simulink model "NewKitchen_demo"  (R2022b)
settings: Solver=FixedStepAuto  StartTime=0  StopTime=3*3600  FixedStep=60  RelTol=1e-3
libraries: dspswit3 x4, dspstat3 x2
settings Model: Creator=u2159176  LastModifiedBy=u2159176

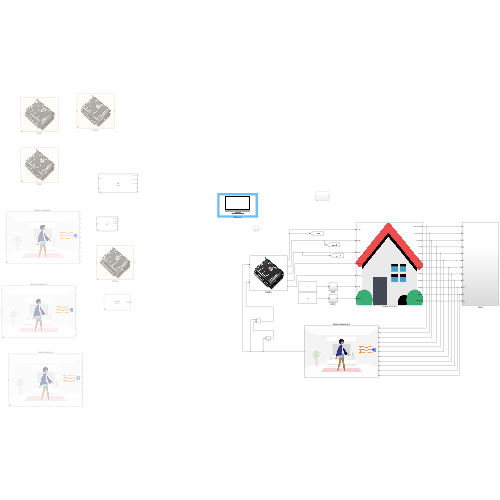
[thumbnail: Simulink's stored preview of the top-level diagram]
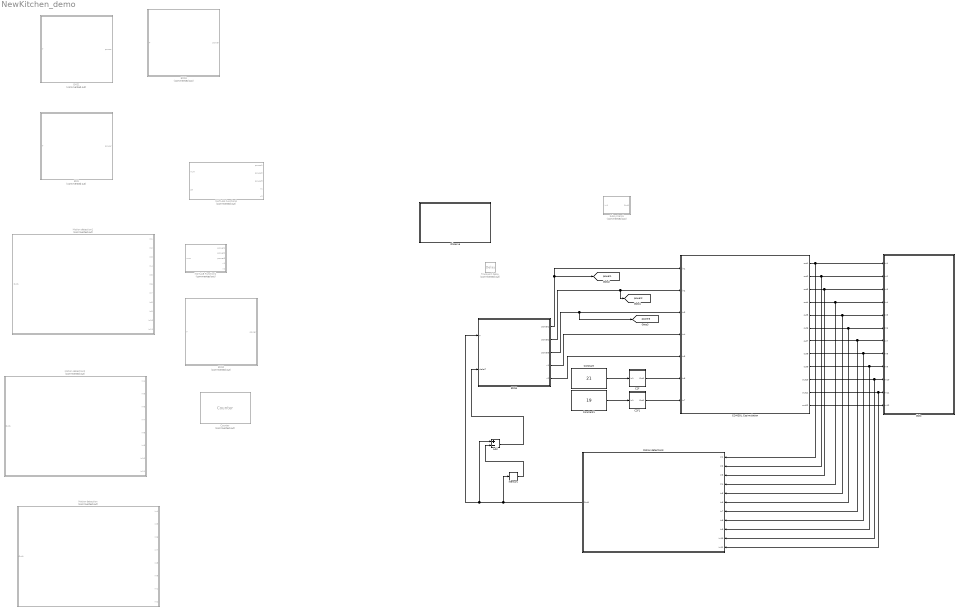
== system NewKitchen_demo ==
  Add : Sum  Inputs=+-
  C2F : Subsystem
  C2F1 : Subsystem
  COMSOL Cosimulation : Subsystem  mask(COMSOL Multiphysics Block){filename=\\brio.ads.warwick.ac.uk\User68\u\u2159176\Desktop\comsol data\ECOS2023\model1201b.fmu, dt=-1}
      mask prompts: dt "Communication step size"
      mask help: COMSOL Multiphysics Block version 6.1
      mask init:
      | if exist('cosimblockinit')==0
      |    error('Can not initialize block. Start COMSOL with Simulink and try again')
      | else
      |     cosimblockinit
      | end
      mask DialogControl bp Prompt: Block Parameters
      mask DialogControl bp Callback: setblockparameters
      mask Display:
      | if isempty(filename)
      |     root = char(java.lang.System.getProperty('cs.root'));
      |     if ~isempty(root)
      |         filename = fullfile(root, 'ext\LiveLink\Simulink\resources\llsimulink_comsol_logo_256.bmp');
      |         if exist(filename, 'file')
      |             im = imread(filename);
      |         end
      |     end
      | end
      | if exist('im', 'var')
      |     image(im)
      | else
      |     disp('COMSOL')
      | end
      | 
      | if exist('labels', 'var')
      |     if isfield(labels, 'in')
      |         for i=1:length(labels.in)
      |             port_label('input', i, labels.in{i})
      |         end
      |     end
      | 
      |     if isfield(labels, 'out')
      |         for i=1:length(labels.out)
      |             port_label('output', i, labels.out{i})
      |         end
      |     end
      | end
  Constant : Constant  Value=21
  Constant1 : Constant  Value=19
  Counter : dspswit3/Counter  Commented=on  Direction=Up  CountEvent=Free running  CounterSize=User defined  MaxCount=480  InitialCount=1  Output=Count  HitValue=1  ResetInput=off  SamplesPerFrame=1  Ts=60  CntDtype=double  HitDtype=Logical
  EMS : Stateflow chart  Commented=on  TreatAsAtomicUnit=on
  EMS1 : Stateflow chart  Commented=on  TreatAsAtomicUnit=on
  EMS2 : Stateflow chart  Commented=on  TreatAsAtomicUnit=on
  EMS3 : Stateflow chart  Commented=on  TreatAsAtomicUnit=on
  EMS4 : Stateflow chart  TreatAsAtomicUnit=on
  Goto : Subsystem
  MATLAB Function1 : MATLAB Function  Commented=on  TreatAsAtomicUnit=on
  MATLAB Function3 : MATLAB Function  Commented=on  TreatAsAtomicUnit=on
  Memory : Memory
  Motion detection : Subsystem  Commented=on
      mask Display: image('\\brio.ads.warwick.ac.uk\User68\u\u2159176\Desktop\comsol data\ECOS2023\tanshen\microwave-sensor.jpg'); % Use "Edit Image" on toolstrip to change.
  Motion detection1 : Subsystem  Commented=on
      mask Display: image('\\brio.ads.warwick.ac.uk\User68\u\u2159176\Desktop\comsol data\ECOS2023\tanshen\microwave-sensor.jpg'); % Use "Edit Image" on toolstrip to change.
  Motion detection2 : Subsystem  Commented=on
      mask Display: image('\\brio.ads.warwick.ac.uk\User68\u\u2159176\Desktop\comsol data\ECOS2023\tanshen\microwave-sensor.jpg'); % Use "Edit Image" on toolstrip to change.
  Motion detection3 : Subsystem
      mask Display: image('\\brio.ads.warwick.ac.uk\User68\u\u2159176\Desktop\comsol data\ECOS2023\tanshen\microwave-sensor.jpg'); % Use "Edit Image" on toolstrip to change.
  Observe : Subsystem
      mask Display: image('\\brio.ads.warwick.ac.uk\User68\u\u2159176\Desktop\comsol data\ECOS2023\tanshen\lcd_display.png'); % Use "Edit Image" on toolstrip to change.
  Subsystem5 : Subsystem  Commented=on
  Transport Delay : TransportDelay  Commented=on
  tag scope: power1=global, power2=global, power3=global
  wires:
  Constant/1 -> C2F/1(In1)
  Constant1/1 -> C2F1/1(In1)
  COMSOL Cosimulation/1(out1) -> Motion detection3/1(In1), Goto/1(In1)
  COMSOL Cosimulation/2(out2) -> Motion detection3/2(In2), Goto/2(In2)
  COMSOL Cosimulation/3(out3) -> Motion detection3/3(In3), Goto/3(In3)
  COMSOL Cosimulation/4(out4) -> Motion detection3/4(In4), Goto/4(In4)
  COMSOL Cosimulation/5(out5) -> Motion detection3/5(In5), Goto/5(In5)
  COMSOL Cosimulation/6(out6) -> Motion detection3/6(In6), Goto/6(In6)
  COMSOL Cosimulation/7(out7) -> Motion detection3/7(In7), Goto/7(In7)
  COMSOL Cosimulation/8(out8) -> Motion detection3/8(In8), Goto/8(In8)
  COMSOL Cosimulation/9(out9) -> Motion detection3/9(In9), Goto/9(In9)
  COMSOL Cosimulation/10(out10) -> Motion detection3/10(In10), Goto/10(In10)
  COMSOL Cosimulation/11(out11) -> Motion detection3/11(In11), Goto/11(In11)
  COMSOL Cosimulation/12(out12) -> Goto/12(In12)
  C2F/1(Out1) -> COMSOL Cosimulation/6(in6)
  C2F1/1(Out1) -> COMSOL Cosimulation/7(in7)
  Motion detection3/1(Out1) -> Add/1, EMS4/1(T), Memory/1
  Memory/1 -> Add/2
  Add/1 -> EMS4/2(deltaT)
  EMS4/1(power1) -> COMSOL Cosimulation/1(in1), [power1]
  EMS4/2(power2) -> [power2], COMSOL Cosimulation/2(in2)
  EMS4/3(power3) -> [power3], COMSOL Cosimulation/3(in3)
  EMS4/4(v1) -> COMSOL Cosimulation/4(in4)
  EMS4/5(v2) -> COMSOL Cosimulation/5(in5)

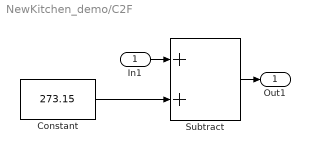
== system NewKitchen_demo/C2F ==
  In1 : Inport
  Constant : Constant  Value=273.15
  Subtract : Sum
  Out1 : Outport
  wires:
  In1/1 -> Subtract/1
  Constant/1 -> Subtract/2
  Subtract/1 -> Out1/1

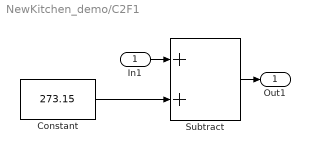
== system NewKitchen_demo/C2F1 ==
  In1 : Inport
  Constant : Constant  Value=273.15
  Subtract : Sum
  Out1 : Outport
  wires:
  Subtract/1 -> Out1/1
  Constant/1 -> Subtract/2
  In1/1 -> Subtract/1

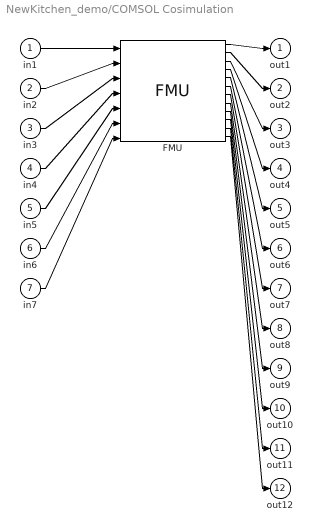
== system NewKitchen_demo/COMSOL Cosimulation ==
  in1 : Inport
  in2 : Inport  Port=2
  in3 : Inport  Port=3
  in4 : Inport  Port=4
  in5 : Inport  Port=5
  in6 : Inport  Port=6
  in7 : Inport  Port=7
  FMU : FMU  FMUName=model1201b.fmu  FMUDebugLogging=on  FMUMode=CoSimulation
      mask Type: demo1122bfor61.mph [Co-Simulation, v2.0]
      mask Display:
      | if (exist([Simulink.fileGenControl('get','CacheFolder') '\slprj\_fmu\ac9248b5f738903d145a6e09f814e397\model1201b\model.png'],'file'))
      |     image([Simulink.fileGenControl('get','CacheFolder') '\slprj\_fmu\ac9248b5f738903d145a6e09f814e397\model1201b\model.png']);
      | else
      |     disp('demo1122bfor61.mph');
      | end
      | port_label('output',1,'comp1.point1');
      | port_label('output',2,'comp1.point2');
      | port_label('output',3,'comp1.point3');
      | port_label('output',4,'comp1.edge1');
      | port_label('output',5,'comp1.edge2');
      | port_label('output',6,'comp1.edge3');
      | port_label('output',7,'comp1.edge4');
      | port_label('output',8,'comp1.edge5');
      | port_label('output',9,'comp1.edge6');
      | port_label('output',10,'comp1.edge7');
      | port_label('output',11,'comp1.edge8');
      | port_label('output',12,'comp1.dom1');
      | port_label('input',1,'P1');
      | port_label('input',2,'P2');
      | port_label('input',3,'P3');
      | port_label('input',4,'V1');
      | port_label('input',5,'V2');
      | port_label('input',6,'Tin');
      | port_label('input',7,'Tout');
  out1 : Outport
  out2 : Outport  Port=2
  out3 : Outport  Port=3
  out4 : Outport  Port=4
  out5 : Outport  Port=5
  out6 : Outport  Port=6
  out7 : Outport  Port=7
  out8 : Outport  Port=8
  out9 : Outport  Port=9
  out10 : Outport  Port=10
  out11 : Outport  Port=11
  out12 : Outport  Port=12
  wires:
  FMU/1 -> out1/1
  FMU/2 -> out2/1
  FMU/3 -> out3/1
  FMU/4 -> out4/1
  FMU/5 -> out5/1
  FMU/6 -> out6/1
  FMU/7 -> out7/1
  FMU/8 -> out8/1
  FMU/9 -> out9/1
  FMU/10 -> out10/1
  FMU/11 -> out11/1
  FMU/12 -> out12/1
  in1/1 -> FMU/1
  in2/1 -> FMU/2
  in3/1 -> FMU/3
  in4/1 -> FMU/4
  in5/1 -> FMU/5
  in6/1 -> FMU/6
  in7/1 -> FMU/7

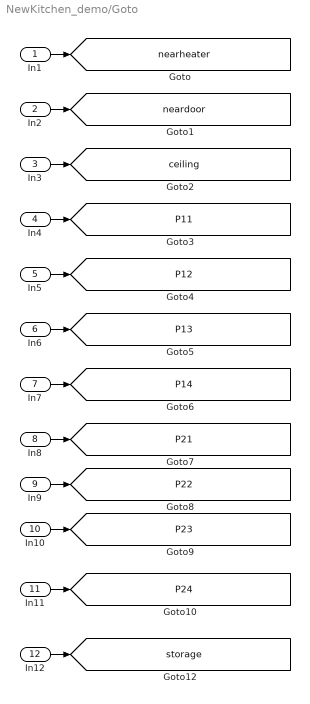
== system NewKitchen_demo/Goto ==
  In1 : Inport
  In2 : Inport  Port=2
  In3 : Inport  Port=3
  In4 : Inport  Port=4
  In5 : Inport  Port=5
  In6 : Inport  Port=6
  In7 : Inport  Port=7
  In8 : Inport  Port=8
  In9 : Inport  Port=9
  In10 : Inport  Port=10
  In11 : Inport  Port=11
  In12 : Inport  Port=12
  tag scope: P11=global, P12=global, P13=global, P14=global, P21=global, P22=global, P23=global, P24=global, ceiling=global, neardoor=global, nearheater=global, storage=global
  wires:
  In2/1 -> [neardoor]
  In10/1 -> [P23]
  In4/1 -> [P11]
  In3/1 -> [ceiling]
  In11/1 -> [P24]
  In8/1 -> [P21]
  In7/1 -> [P14]
  In5/1 -> [P12]
  In6/1 -> [P13]
  In1/1 -> [nearheater]
  In9/1 -> [P22]
  In12/1 -> [storage]

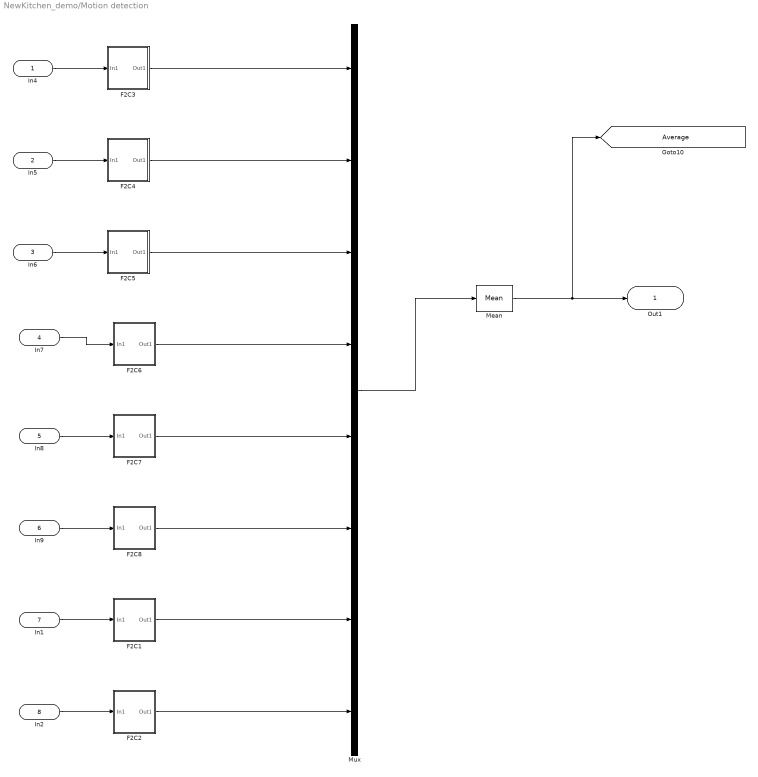
== system NewKitchen_demo/Motion detection ==
  In4 : Inport
  In5 : Inport  Port=2
  In6 : Inport  Port=3
  In7 : Inport  Port=4
  In8 : Inport  Port=5
  In9 : Inport  Port=6
  In1 : Inport  Port=7
  In2 : Inport  Port=8
  F2C1 : Subsystem
  F2C2 : Subsystem
  F2C3 : Subsystem
  F2C4 : Subsystem
  F2C5 : Subsystem
  F2C6 : Subsystem
  F2C7 : Subsystem
  F2C8 : Subsystem
  Mean : dspstat3/Mean  run=off  InputProcessing=Columns as channels (frame based)  reset_popup=None  directionMode=Each column  dimension=1  roiEnable=off  roiType=Rectangles  roiPortion=Entire ROI  roiOutput=Individual statistics for each ROI  roiFlag=off  roundingMode=Floor  overflowMode=off  outputDataTypeStr=Inherit: Same as accumulator  outputMin=[]  outputMax=[]  outputLastDataTypeStr=Inherit: Same as accumulator
  Mux : Mux  Inputs=8
  Out1 : Outport
  tag scope: Average=global
  wires:
  In4/1 -> F2C3/1(In1)
  In5/1 -> F2C4/1(In1)
  In6/1 -> F2C5/1(In1)
  In7/1 -> F2C6/1(In1)
  In8/1 -> F2C7/1(In1)
  In9/1 -> F2C8/1(In1)
  Mean/1 -> [Average], Out1/1
  Mux/1 -> Mean/1
  F2C3/1(Out1) -> Mux/1
  F2C4/1(Out1) -> Mux/2
  F2C5/1(Out1) -> Mux/3
  F2C6/1(Out1) -> Mux/4
  F2C7/1(Out1) -> Mux/5
  F2C8/1(Out1) -> Mux/6
  F2C1/1(Out1) -> Mux/7
  In1/1 -> F2C1/1(In1)
  In2/1 -> F2C2/1(In1)
  F2C2/1(Out1) -> Mux/8

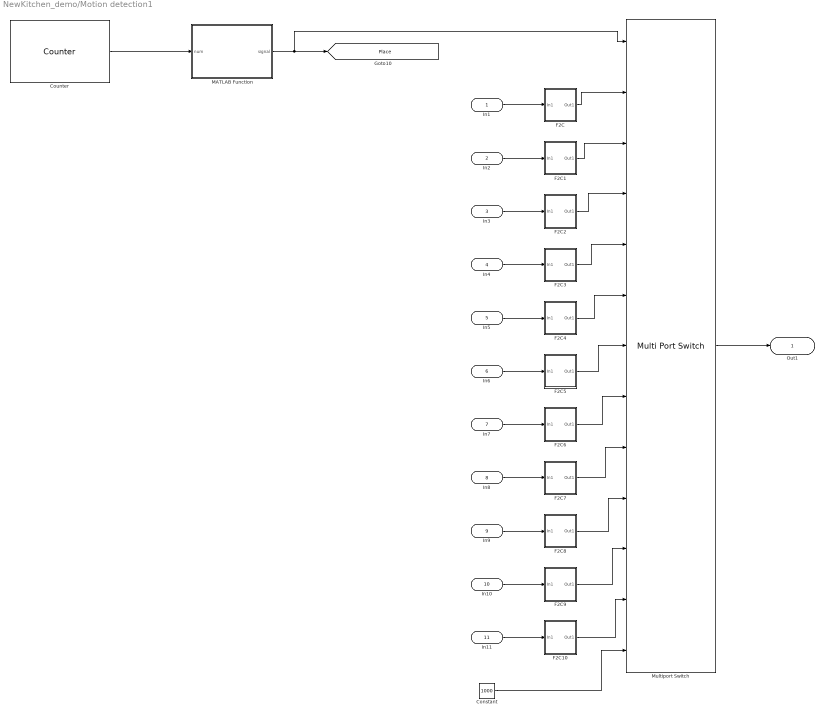
== system NewKitchen_demo/Motion detection1 ==
  In1 : Inport
  In2 : Inport  Port=2
  In3 : Inport  Port=3
  In4 : Inport  Port=4
  In5 : Inport  Port=5
  In6 : Inport  Port=6
  In7 : Inport  Port=7
  In8 : Inport  Port=8
  In9 : Inport  Port=9
  In10 : Inport  Port=10
  In11 : Inport  Port=11
  Constant : Constant  Value=1000
  Counter : dspswit3/Counter  Direction=Up  CountEvent=Free running  CounterSize=User defined  MaxCount=480  InitialCount=1  Output=Count  HitValue=1  ResetInput=off  SamplesPerFrame=1  Ts=60  CntDtype=double  HitDtype=Logical
  F2C : Subsystem
  F2C1 : Subsystem
  F2C10 : Subsystem
  F2C2 : Subsystem
  F2C3 : Subsystem
  F2C4 : Subsystem
  F2C5 : Subsystem
  F2C6 : Subsystem
  F2C7 : Subsystem
  F2C8 : Subsystem
  F2C9 : Subsystem
  MATLAB Function : MATLAB Function  TreatAsAtomicUnit=on
  Multiport Switch : MultiPortSwitch  Inputs=12  SaturateOnIntegerOverflow=off  InputSameDT=off
  Out1 : Outport
  tag scope: Place=global
  wires:
  Constant/1 -> Multiport Switch/13
  MATLAB Function/1(signal) -> [Place], Multiport Switch/1
  Counter/1 -> MATLAB Function/1(num)
  Multiport Switch/1 -> Out1/1
  In11/1 -> F2C10/1(In1)
  In10/1 -> F2C9/1(In1)
  In9/1 -> F2C8/1(In1)
  In8/1 -> F2C7/1(In1)
  In7/1 -> F2C6/1(In1)
  In6/1 -> F2C5/1(In1)
  In5/1 -> F2C4/1(In1)
  In4/1 -> F2C3/1(In1)
  In3/1 -> F2C2/1(In1)
  In2/1 -> F2C1/1(In1)
  In1/1 -> F2C/1(In1)
  F2C10/1(Out1) -> Multiport Switch/12
  F2C9/1(Out1) -> Multiport Switch/11
  F2C8/1(Out1) -> Multiport Switch/10
  F2C7/1(Out1) -> Multiport Switch/9
  F2C6/1(Out1) -> Multiport Switch/8
  F2C5/1(Out1) -> Multiport Switch/7
  F2C4/1(Out1) -> Multiport Switch/6
  F2C3/1(Out1) -> Multiport Switch/5
  F2C2/1(Out1) -> Multiport Switch/4
  F2C1/1(Out1) -> Multiport Switch/3
  F2C/1(Out1) -> Multiport Switch/2

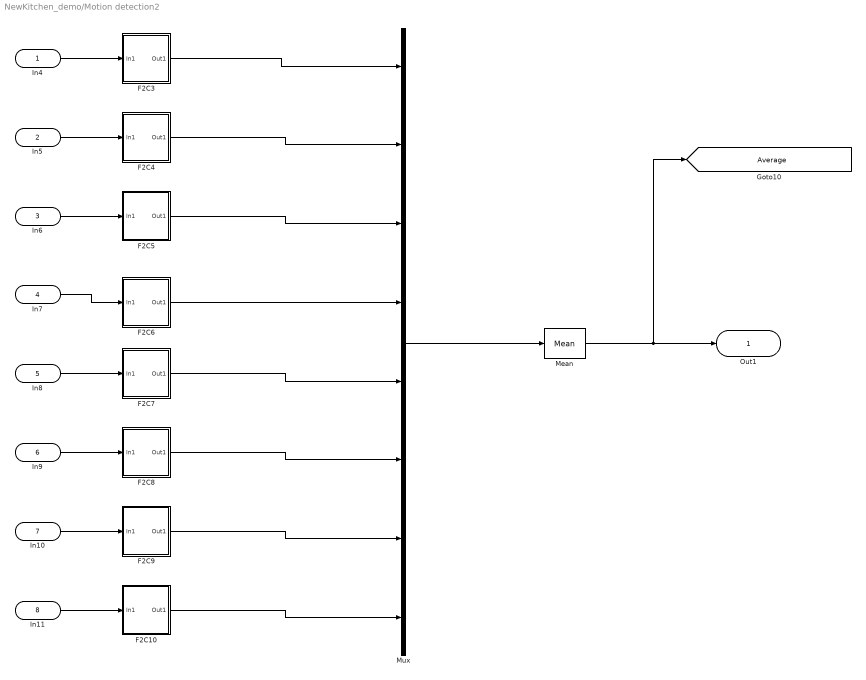
== system NewKitchen_demo/Motion detection2 ==
  In4 : Inport
  In5 : Inport  Port=2
  In6 : Inport  Port=3
  In7 : Inport  Port=4
  In8 : Inport  Port=5
  In9 : Inport  Port=6
  In10 : Inport  Port=7
  In11 : Inport  Port=8
  F2C10 : Subsystem
  F2C3 : Subsystem
  F2C4 : Subsystem
  F2C5 : Subsystem
  F2C6 : Subsystem
  F2C7 : Subsystem
  F2C8 : Subsystem
  F2C9 : Subsystem
  Mean : dspstat3/Mean  run=off  InputProcessing=Columns as channels (frame based)  reset_popup=None  directionMode=Each column  dimension=1  roiEnable=off  roiType=Rectangles  roiPortion=Entire ROI  roiOutput=Individual statistics for each ROI  roiFlag=off  roundingMode=Floor  overflowMode=off  outputDataTypeStr=Inherit: Same as accumulator  outputMin=[]  outputMax=[]  outputLastDataTypeStr=Inherit: Same as accumulator
  Mux : Mux  Inputs=8
  Out1 : Outport
  tag scope: Average=global
  wires:
  F2C10/1(Out1) -> Mux/8
  F2C9/1(Out1) -> Mux/7
  F2C8/1(Out1) -> Mux/6
  F2C7/1(Out1) -> Mux/5
  F2C6/1(Out1) -> Mux/4
  F2C5/1(Out1) -> Mux/3
  F2C4/1(Out1) -> Mux/2
  F2C3/1(Out1) -> Mux/1
  Mux/1 -> Mean/1
  Mean/1 -> Out1/1, [Average]
  In11/1 -> F2C10/1(In1)
  In10/1 -> F2C9/1(In1)
  In9/1 -> F2C8/1(In1)
  In8/1 -> F2C7/1(In1)
  In7/1 -> F2C6/1(In1)
  In6/1 -> F2C5/1(In1)
  In5/1 -> F2C4/1(In1)
  In4/1 -> F2C3/1(In1)

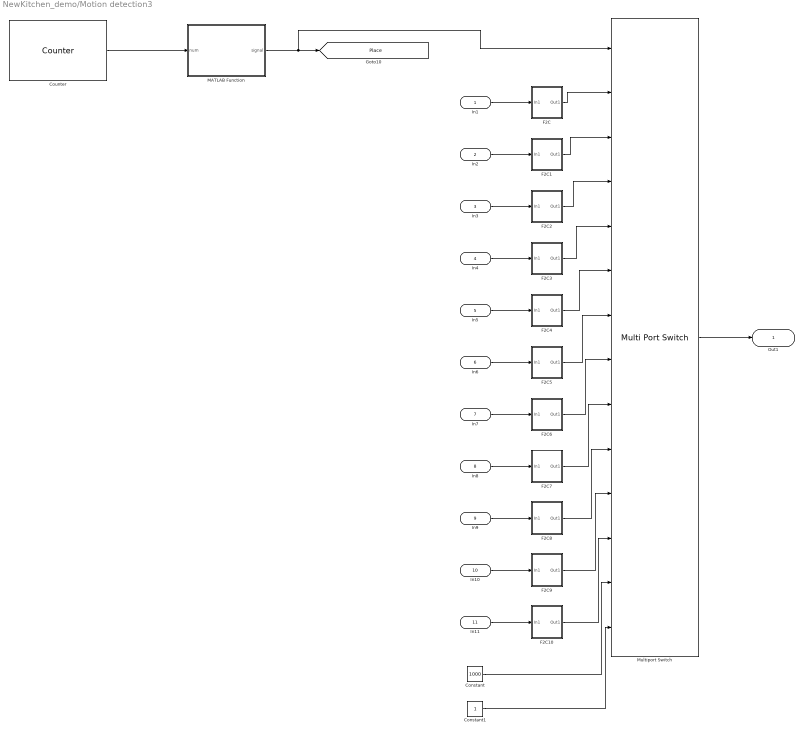
== system NewKitchen_demo/Motion detection3 ==
  In1 : Inport
  In2 : Inport  Port=2
  In3 : Inport  Port=3
  In4 : Inport  Port=4
  In5 : Inport  Port=5
  In6 : Inport  Port=6
  In7 : Inport  Port=7
  In8 : Inport  Port=8
  In9 : Inport  Port=9
  In10 : Inport  Port=10
  In11 : Inport  Port=11
  Constant : Constant  Value=1000
  Constant1 : Constant
  Counter : dspswit3/Counter  Direction=Up  CountEvent=Free running  CounterSize=User defined  MaxCount=480  InitialCount=1  Output=Count  HitValue=1  ResetInput=off  SamplesPerFrame=1  Ts=60  CntDtype=double  HitDtype=Logical
  F2C : Subsystem
  F2C1 : Subsystem
  F2C10 : Subsystem
  F2C2 : Subsystem
  F2C3 : Subsystem
  F2C4 : Subsystem
  F2C5 : Subsystem
  F2C6 : Subsystem
  F2C7 : Subsystem
  F2C8 : Subsystem
  F2C9 : Subsystem
  MATLAB Function : MATLAB Function  TreatAsAtomicUnit=on
  Multiport Switch : MultiPortSwitch  Inputs=13  SaturateOnIntegerOverflow=off  InputSameDT=off
  Out1 : Outport
  tag scope: Place=global
  wires:
  F2C/1(Out1) -> Multiport Switch/2
  F2C1/1(Out1) -> Multiport Switch/3
  F2C2/1(Out1) -> Multiport Switch/4
  F2C3/1(Out1) -> Multiport Switch/5
  F2C4/1(Out1) -> Multiport Switch/6
  F2C5/1(Out1) -> Multiport Switch/7
  F2C6/1(Out1) -> Multiport Switch/8
  F2C7/1(Out1) -> Multiport Switch/9
  F2C8/1(Out1) -> Multiport Switch/10
  F2C9/1(Out1) -> Multiport Switch/11
  F2C10/1(Out1) -> Multiport Switch/12
  In1/1 -> F2C/1(In1)
  In2/1 -> F2C1/1(In1)
  In3/1 -> F2C2/1(In1)
  In4/1 -> F2C3/1(In1)
  In5/1 -> F2C4/1(In1)
  In6/1 -> F2C5/1(In1)
  In7/1 -> F2C6/1(In1)
  In8/1 -> F2C7/1(In1)
  In9/1 -> F2C8/1(In1)
  In10/1 -> F2C9/1(In1)
  In11/1 -> F2C10/1(In1)
  Multiport Switch/1 -> Out1/1
  Counter/1 -> MATLAB Function/1(num)
  MATLAB Function/1(signal) -> Multiport Switch/1, [Place]
  Constant/1 -> Multiport Switch/13
  Constant1/1 -> Multiport Switch/14

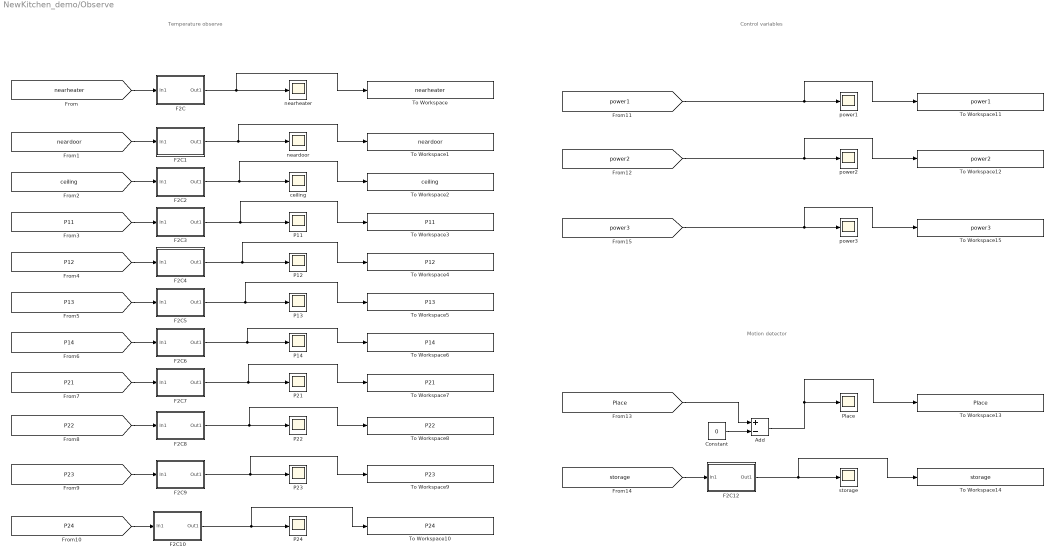
== system NewKitchen_demo/Observe ==
  note: Temperature observe
  note: Control variables
  note: Motion detector
  Add : Sum  Inputs=+-
  Constant : Constant  Value=0
  F2C : Subsystem
  F2C1 : Subsystem
  F2C10 : Subsystem
  F2C12 : Subsystem
  F2C2 : Subsystem
  F2C3 : Subsystem
  F2C4 : Subsystem
  F2C5 : Subsystem
  F2C6 : Subsystem
  F2C7 : Subsystem
  F2C8 : Subsystem
  F2C9 : Subsystem
  P{11..14,21..24} (8 alike) : Scope
  Place : Scope
  To Workspace : ToWorkspace  VariableName=nearheater  SampleTime=-1
  To Workspace1 : ToWorkspace  VariableName=neardoor  SampleTime=-1
  To Workspace10 : ToWorkspace  VariableName=P24  SampleTime=-1
  To Workspace11 : ToWorkspace  VariableName=power1  SampleTime=-1
  To Workspace12 : ToWorkspace  VariableName=power2  SampleTime=-1
  To Workspace13 : ToWorkspace  VariableName=Place  SampleTime=-1
  To Workspace14 : ToWorkspace  VariableName=storage  SampleTime=-1
  To Workspace15 : ToWorkspace  VariableName=power3  SampleTime=-1
  To Workspace2 : ToWorkspace  VariableName=ceiling  SampleTime=-1
  To Workspace3 : ToWorkspace  VariableName=P11  SampleTime=-1
  To Workspace4 : ToWorkspace  VariableName=P12  SampleTime=-1
  To Workspace5 : ToWorkspace  VariableName=P13  SampleTime=-1
  To Workspace6 : ToWorkspace  VariableName=P14  SampleTime=-1
  To Workspace7 : ToWorkspace  VariableName=P21  SampleTime=-1
  To Workspace8 : ToWorkspace  VariableName=P22  SampleTime=-1
  To Workspace9 : ToWorkspace  VariableName=P23  SampleTime=-1
  ceiling : Scope
  neardoor : Scope
  nearheater : Scope
  power1 : Scope
  power2 : Scope
  power3 : Scope
  storage : Scope
  wires:
  [nearheater] -> F2C/1(In1)
  F2C/1(Out1) -> To Workspace/1, nearheater/1
  [neardoor] -> F2C1/1(In1)
  F2C1/1(Out1) -> To Workspace1/1, neardoor/1
  [ceiling] -> F2C2/1(In1)
  F2C2/1(Out1) -> To Workspace2/1, ceiling/1
  [P11] -> F2C3/1(In1)
  F2C3/1(Out1) -> To Workspace3/1, P11/1
  [P12] -> F2C4/1(In1)
  F2C4/1(Out1) -> To Workspace4/1, P12/1
  [P13] -> F2C5/1(In1)
  F2C5/1(Out1) -> To Workspace5/1, P13/1
  [P14] -> F2C6/1(In1)
  F2C6/1(Out1) -> To Workspace6/1, P14/1
  [P21] -> F2C7/1(In1)
  F2C7/1(Out1) -> To Workspace7/1, P21/1
  [P22] -> F2C8/1(In1)
  F2C8/1(Out1) -> To Workspace8/1, P22/1
  [P23] -> F2C9/1(In1)
  F2C9/1(Out1) -> To Workspace9/1, P23/1
  [P24] -> F2C10/1(In1)
  [power1] -> To Workspace11/1, power1/1
  F2C10/1(Out1) -> To Workspace10/1, P24/1
  F2C12/1(Out1) -> storage/1, To Workspace14/1
  [storage] -> F2C12/1(In1)
  [power2] -> power2/1, To Workspace12/1
  [power3] -> To Workspace15/1, power3/1
  Constant/1 -> Add/2
  [Place] -> Add/1
  Add/1 -> To Workspace13/1, Place/1

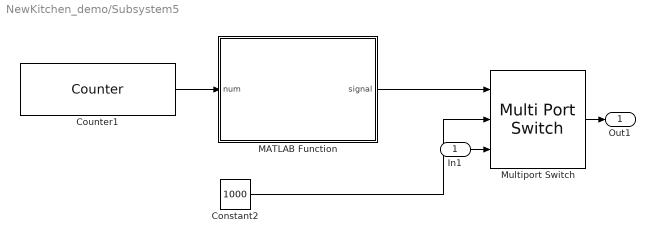
== system NewKitchen_demo/Subsystem5 ==
  In1 : Inport
  Constant2 : Constant  Value=1000
  Counter1 : dspswit3/Counter  Direction=Up  CountEvent=Free running  CounterSize=User defined  MaxCount=480  InitialCount=1  Output=Count  HitValue=1  ResetInput=off  SamplesPerFrame=1  Ts=60  CntDtype=double  HitDtype=Logical
  MATLAB Function : MATLAB Function  TreatAsAtomicUnit=on
  Multiport Switch : MultiPortSwitch  Inputs=2  SaturateOnIntegerOverflow=off  InputSameDT=off
  Out1 : Outport
  wires:
  Multiport Switch/1 -> Out1/1
  Constant2/1 -> Multiport Switch/2
  MATLAB Function/1(signal) -> Multiport Switch/1
  In1/1 -> Multiport Switch/3
  Counter1/1 -> MATLAB Function/1(num)

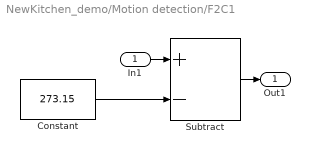
== system NewKitchen_demo/Motion detection/F2C1 ==
  In1 : Inport
  Constant : Constant  Value=273.15
  Subtract : Sum  Inputs=+-
  Out1 : Outport
  wires:
  Subtract/1 -> Out1/1
  Constant/1 -> Subtract/2
  In1/1 -> Subtract/1

== system NewKitchen_demo/Motion detection/F2C2 ==
  In1 : Inport
  Constant : Constant  Value=273.15
  Subtract : Sum  Inputs=+-
  Out1 : Outport
  wires:
  In1/1 -> Subtract/1
  Constant/1 -> Subtract/2
  Subtract/1 -> Out1/1

== system NewKitchen_demo/Motion detection/F2C3 ==
  In1 : Inport
  Constant : Constant  Value=273.15
  Subtract : Sum  Inputs=+-
  Out1 : Outport
  wires:
  Subtract/1 -> Out1/1
  Constant/1 -> Subtract/2
  In1/1 -> Subtract/1

== system NewKitchen_demo/Motion detection/F2C4 ==
  In1 : Inport
  Constant : Constant  Value=273.15
  Subtract : Sum  Inputs=+-
  Out1 : Outport
  wires:
  In1/1 -> Subtract/1
  Constant/1 -> Subtract/2
  Subtract/1 -> Out1/1

== system NewKitchen_demo/Motion detection/F2C5 ==
  In1 : Inport
  Constant : Constant  Value=273.15
  Subtract : Sum  Inputs=+-
  Out1 : Outport
  wires:
  Subtract/1 -> Out1/1
  Constant/1 -> Subtract/2
  In1/1 -> Subtract/1

== system NewKitchen_demo/Motion detection/F2C6 ==
  In1 : Inport
  Constant : Constant  Value=273.15
  Subtract : Sum  Inputs=+-
  Out1 : Outport
  wires:
  In1/1 -> Subtract/1
  Constant/1 -> Subtract/2
  Subtract/1 -> Out1/1

== system NewKitchen_demo/Motion detection/F2C7 ==
  In1 : Inport
  Constant : Constant  Value=273.15
  Subtract : Sum  Inputs=+-
  Out1 : Outport
  wires:
  Subtract/1 -> Out1/1
  Constant/1 -> Subtract/2
  In1/1 -> Subtract/1

== system NewKitchen_demo/Motion detection/F2C8 ==
  In1 : Inport
  Constant : Constant  Value=273.15
  Subtract : Sum  Inputs=+-
  Out1 : Outport
  wires:
  In1/1 -> Subtract/1
  Constant/1 -> Subtract/2
  Subtract/1 -> Out1/1

== system NewKitchen_demo/Motion detection1/F2C ==
  In1 : Inport
  Constant : Constant  Value=273.15
  Subtract : Sum  Inputs=+-
  Out1 : Outport
  wires:
  Subtract/1 -> Out1/1
  Constant/1 -> Subtract/2
  In1/1 -> Subtract/1

== system NewKitchen_demo/Motion detection1/F2C1 ==
  In1 : Inport
  Constant : Constant  Value=273.15
  Subtract : Sum  Inputs=+-
  Out1 : Outport
  wires:
  In1/1 -> Subtract/1
  Constant/1 -> Subtract/2
  Subtract/1 -> Out1/1

== system NewKitchen_demo/Motion detection1/F2C10 ==
  In1 : Inport
  Constant : Constant  Value=273.15
  Subtract : Sum  Inputs=+-
  Out1 : Outport
  wires:
  Subtract/1 -> Out1/1
  Constant/1 -> Subtract/2
  In1/1 -> Subtract/1

== system NewKitchen_demo/Motion detection1/F2C2 ==
  In1 : Inport
  Constant : Constant  Value=273.15
  Subtract : Sum  Inputs=+-
  Out1 : Outport
  wires:
  Subtract/1 -> Out1/1
  Constant/1 -> Subtract/2
  In1/1 -> Subtract/1

== system NewKitchen_demo/Motion detection1/F2C3 ==
  In1 : Inport
  Constant : Constant  Value=273.15
  Subtract : Sum  Inputs=+-
  Out1 : Outport
  wires:
  In1/1 -> Subtract/1
  Constant/1 -> Subtract/2
  Subtract/1 -> Out1/1

== system NewKitchen_demo/Motion detection1/F2C4 ==
  In1 : Inport
  Constant : Constant  Value=273.15
  Subtract : Sum  Inputs=+-
  Out1 : Outport
  wires:
  Subtract/1 -> Out1/1
  Constant/1 -> Subtract/2
  In1/1 -> Subtract/1

== system NewKitchen_demo/Motion detection1/F2C5 ==
  In1 : Inport
  Constant : Constant  Value=273.15
  Subtract : Sum  Inputs=+-
  Out1 : Outport
  wires:
  In1/1 -> Subtract/1
  Constant/1 -> Subtract/2
  Subtract/1 -> Out1/1

== system NewKitchen_demo/Motion detection1/F2C6 ==
  In1 : Inport
  Constant : Constant  Value=273.15
  Subtract : Sum  Inputs=+-
  Out1 : Outport
  wires:
  Subtract/1 -> Out1/1
  Constant/1 -> Subtract/2
  In1/1 -> Subtract/1

== system NewKitchen_demo/Motion detection1/F2C7 ==
  In1 : Inport
  Constant : Constant  Value=273.15
  Subtract : Sum  Inputs=+-
  Out1 : Outport
  wires:
  In1/1 -> Subtract/1
  Constant/1 -> Subtract/2
  Subtract/1 -> Out1/1

== system NewKitchen_demo/Motion detection1/F2C8 ==
  In1 : Inport
  Constant : Constant  Value=273.15
  Subtract : Sum  Inputs=+-
  Out1 : Outport
  wires:
  Subtract/1 -> Out1/1
  Constant/1 -> Subtract/2
  In1/1 -> Subtract/1

== system NewKitchen_demo/Motion detection1/F2C9 ==
  In1 : Inport
  Constant : Constant  Value=273.15
  Subtract : Sum  Inputs=+-
  Out1 : Outport
  wires:
  In1/1 -> Subtract/1
  Constant/1 -> Subtract/2
  Subtract/1 -> Out1/1

== system NewKitchen_demo/Motion detection2/F2C10 ==
  In1 : Inport
  Constant : Constant  Value=273.15
  Subtract : Sum  Inputs=+-
  Out1 : Outport
  wires:
  Subtract/1 -> Out1/1
  Constant/1 -> Subtract/2
  In1/1 -> Subtract/1

== system NewKitchen_demo/Motion detection2/F2C3 ==
  In1 : Inport
  Constant : Constant  Value=273.15
  Subtract : Sum  Inputs=+-
  Out1 : Outport
  wires:
  In1/1 -> Subtract/1
  Constant/1 -> Subtract/2
  Subtract/1 -> Out1/1

== system NewKitchen_demo/Motion detection2/F2C4 ==
  In1 : Inport
  Constant : Constant  Value=273.15
  Subtract : Sum  Inputs=+-
  Out1 : Outport
  wires:
  Subtract/1 -> Out1/1
  Constant/1 -> Subtract/2
  In1/1 -> Subtract/1

== system NewKitchen_demo/Motion detection2/F2C5 ==
  In1 : Inport
  Constant : Constant  Value=273.15
  Subtract : Sum  Inputs=+-
  Out1 : Outport
  wires:
  In1/1 -> Subtract/1
  Constant/1 -> Subtract/2
  Subtract/1 -> Out1/1

== system NewKitchen_demo/Motion detection2/F2C6 ==
  In1 : Inport
  Constant : Constant  Value=273.15
  Subtract : Sum  Inputs=+-
  Out1 : Outport
  wires:
  Subtract/1 -> Out1/1
  Constant/1 -> Subtract/2
  In1/1 -> Subtract/1

== system NewKitchen_demo/Motion detection2/F2C7 ==
  In1 : Inport
  Constant : Constant  Value=273.15
  Subtract : Sum  Inputs=+-
  Out1 : Outport
  wires:
  In1/1 -> Subtract/1
  Constant/1 -> Subtract/2
  Subtract/1 -> Out1/1

== system NewKitchen_demo/Motion detection2/F2C8 ==
  In1 : Inport
  Constant : Constant  Value=273.15
  Subtract : Sum  Inputs=+-
  Out1 : Outport
  wires:
  Subtract/1 -> Out1/1
  Constant/1 -> Subtract/2
  In1/1 -> Subtract/1

== system NewKitchen_demo/Motion detection2/F2C9 ==
  In1 : Inport
  Constant : Constant  Value=273.15
  Subtract : Sum  Inputs=+-
  Out1 : Outport
  wires:
  In1/1 -> Subtract/1
  Constant/1 -> Subtract/2
  Subtract/1 -> Out1/1

== system NewKitchen_demo/Motion detection3/F2C ==
  In1 : Inport
  Constant : Constant  Value=273.15
  Subtract : Sum  Inputs=+-
  Out1 : Outport
  wires:
  In1/1 -> Subtract/1
  Constant/1 -> Subtract/2
  Subtract/1 -> Out1/1

== system NewKitchen_demo/Motion detection3/F2C1 ==
  In1 : Inport
  Constant : Constant  Value=273.15
  Subtract : Sum  Inputs=+-
  Out1 : Outport
  wires:
  Subtract/1 -> Out1/1
  Constant/1 -> Subtract/2
  In1/1 -> Subtract/1

== system NewKitchen_demo/Motion detection3/F2C10 ==
  In1 : Inport
  Constant : Constant  Value=273.15
  Subtract : Sum  Inputs=+-
  Out1 : Outport
  wires:
  In1/1 -> Subtract/1
  Constant/1 -> Subtract/2
  Subtract/1 -> Out1/1

== system NewKitchen_demo/Motion detection3/F2C2 ==
  In1 : Inport
  Constant : Constant  Value=273.15
  Subtract : Sum  Inputs=+-
  Out1 : Outport
  wires:
  In1/1 -> Subtract/1
  Constant/1 -> Subtract/2
  Subtract/1 -> Out1/1

== system NewKitchen_demo/Motion detection3/F2C3 ==
  In1 : Inport
  Constant : Constant  Value=273.15
  Subtract : Sum  Inputs=+-
  Out1 : Outport
  wires:
  Subtract/1 -> Out1/1
  Constant/1 -> Subtract/2
  In1/1 -> Subtract/1

== system NewKitchen_demo/Motion detection3/F2C4 ==
  In1 : Inport
  Constant : Constant  Value=273.15
  Subtract : Sum  Inputs=+-
  Out1 : Outport
  wires:
  In1/1 -> Subtract/1
  Constant/1 -> Subtract/2
  Subtract/1 -> Out1/1

== system NewKitchen_demo/Motion detection3/F2C5 ==
  In1 : Inport
  Constant : Constant  Value=273.15
  Subtract : Sum  Inputs=+-
  Out1 : Outport
  wires:
  Subtract/1 -> Out1/1
  Constant/1 -> Subtract/2
  In1/1 -> Subtract/1

== system NewKitchen_demo/Motion detection3/F2C6 ==
  In1 : Inport
  Constant : Constant  Value=273.15
  Subtract : Sum  Inputs=+-
  Out1 : Outport
  wires:
  In1/1 -> Subtract/1
  Constant/1 -> Subtract/2
  Subtract/1 -> Out1/1

== system NewKitchen_demo/Motion detection3/F2C7 ==
  In1 : Inport
  Constant : Constant  Value=273.15
  Subtract : Sum  Inputs=+-
  Out1 : Outport
  wires:
  Subtract/1 -> Out1/1
  Constant/1 -> Subtract/2
  In1/1 -> Subtract/1

== system NewKitchen_demo/Motion detection3/F2C8 ==
  In1 : Inport
  Constant : Constant  Value=273.15
  Subtract : Sum  Inputs=+-
  Out1 : Outport
  wires:
  In1/1 -> Subtract/1
  Constant/1 -> Subtract/2
  Subtract/1 -> Out1/1

== system NewKitchen_demo/Motion detection3/F2C9 ==
  In1 : Inport
  Constant : Constant  Value=273.15
  Subtract : Sum  Inputs=+-
  Out1 : Outport
  wires:
  Subtract/1 -> Out1/1
  Constant/1 -> Subtract/2
  In1/1 -> Subtract/1

== system NewKitchen_demo/Observe/F2C ==
  In1 : Inport
  Constant : Constant  Value=273.15
  Subtract : Sum  Inputs=+-
  Out1 : Outport
  wires:
  In1/1 -> Subtract/1
  Constant/1 -> Subtract/2
  Subtract/1 -> Out1/1

== system NewKitchen_demo/Observe/F2C1 ==
  In1 : Inport
  Constant : Constant  Value=273.15
  Subtract : Sum  Inputs=+-
  Out1 : Outport
  wires:
  Subtract/1 -> Out1/1
  Constant/1 -> Subtract/2
  In1/1 -> Subtract/1

== system NewKitchen_demo/Observe/F2C10 ==
  In1 : Inport
  Constant : Constant  Value=273.15
  Subtract : Sum  Inputs=+-
  Out1 : Outport
  wires:
  In1/1 -> Subtract/1
  Constant/1 -> Subtract/2
  Subtract/1 -> Out1/1

== system NewKitchen_demo/Observe/F2C12 ==
  In1 : Inport
  Constant : Constant  Value=273.15
  Subtract : Sum  Inputs=+-
  Out1 : Outport
  wires:
  In1/1 -> Subtract/1
  Constant/1 -> Subtract/2
  Subtract/1 -> Out1/1

== system NewKitchen_demo/Observe/F2C2 ==
  In1 : Inport
  Constant : Constant  Value=273.15
  Subtract : Sum  Inputs=+-
  Out1 : Outport
  wires:
  In1/1 -> Subtract/1
  Constant/1 -> Subtract/2
  Subtract/1 -> Out1/1

== system NewKitchen_demo/Observe/F2C3 ==
  In1 : Inport
  Constant : Constant  Value=273.15
  Subtract : Sum  Inputs=+-
  Out1 : Outport
  wires:
  Subtract/1 -> Out1/1
  Constant/1 -> Subtract/2
  In1/1 -> Subtract/1

== system NewKitchen_demo/Observe/F2C4 ==
  In1 : Inport
  Constant : Constant  Value=273.15
  Subtract : Sum  Inputs=+-
  Out1 : Outport
  wires:
  In1/1 -> Subtract/1
  Constant/1 -> Subtract/2
  Subtract/1 -> Out1/1

== system NewKitchen_demo/Observe/F2C5 ==
  In1 : Inport
  Constant : Constant  Value=273.15
  Subtract : Sum  Inputs=+-
  Out1 : Outport
  wires:
  Subtract/1 -> Out1/1
  Constant/1 -> Subtract/2
  In1/1 -> Subtract/1

== system NewKitchen_demo/Observe/F2C6 ==
  In1 : Inport
  Constant : Constant  Value=273.15
  Subtract : Sum  Inputs=+-
  Out1 : Outport
  wires:
  In1/1 -> Subtract/1
  Constant/1 -> Subtract/2
  Subtract/1 -> Out1/1

== system NewKitchen_demo/Observe/F2C7 ==
  In1 : Inport
  Constant : Constant  Value=273.15
  Subtract : Sum  Inputs=+-
  Out1 : Outport
  wires:
  Subtract/1 -> Out1/1
  Constant/1 -> Subtract/2
  In1/1 -> Subtract/1

== system NewKitchen_demo/Observe/F2C8 ==
  In1 : Inport
  Constant : Constant  Value=273.15
  Subtract : Sum  Inputs=+-
  Out1 : Outport
  wires:
  In1/1 -> Subtract/1
  Constant/1 -> Subtract/2
  Subtract/1 -> Out1/1

== system NewKitchen_demo/Observe/F2C9 ==
  In1 : Inport
  Constant : Constant  Value=273.15
  Subtract : Sum  Inputs=+-
  Out1 : Outport
  wires:
  Subtract/1 -> Out1/1
  Constant/1 -> Subtract/2
  In1/1 -> Subtract/1

== stateflow chart NewKitchen_demo/EMS ==
  state OFF_Mode
    during:
    power = 0;
  state ON_Mode
    state Mode1
      during:
      power=3300;
    state Mode2
      during:
      power=1100;
    (default) -> Mode1
    Mode1 -> Mode2 : [T>21.6]
  (default) -> (junction 1)
  (junction 1) -> OFF_Mode [order 1] : [T>=25]
  (junction 1) -> ON_Mode [order 2]
  OFF_Mode -> ON_Mode : [T<21]
  ON_Mode -> OFF_Mode : [T>=22]
  data: T input; power output

== matlab function NewKitchen_demo/MATLAB Function3 ==
  data: power1 output; power2 output; power3 output; num input; v1 output; v2 output; CT input
function [power1,power2,power3,v1,v2] = motion(num,CT)
    
%     N = ceil(num/30); 

    deltaT = num - 23;
    

    if num < 10
        power1 = 1000;
        power2 = 1000;
        power3 = 1000;
        v1 = 0;
        v2 = 0;
    else
        if deltaT <= -0.5
            if CT <= 0.09
                power1 = 1000;
                power2 = 1000;
                power3 = 1000;
                v1 = 2;
                v2 = 1;
            else
                power1 = 0;
                power2 = 0;
                power3 = 0;
                v1 = 2;
                v2 = 1;
            end
        else
            if deltaT <= 0.5
                if CT <= 0.06
                    power1 = 1000;
                    power2 = 1000;
                    power3 = 0;
                    v1 = 2;
                    v2 = 1;
                else
                    power1 = 0;
                    power2 = 0;
                    power3 = 0;
                    v1 = 2;
                    v2 = 1;
                end
            else
                if deltaT <= 1
                    if CT <= 0.03
                        power1 = 1000;
                        power2 = 0;
                        power3 = 0;
                        v1 = 2;
                        v2 = 1;
                    else
                        power1 = 0;
                        power2 = 0;
                        power3 = 0;
                        v1 = 2;
                        v2 = 1;
                    end
                else
                    power1 = 0;
                    power2 = 0;
                    power3 = 0;
                    v1 = 0;
                    v2 = 0;
                end
            end
        end     
    end
end

%     if deltaT <= -0.5
%         power1 = 1000;
%         power2 = 1000;
%         power3 = 1000;
%         v1 = 2;
%         v2 = 1;
%     else
% 
%         if deltaT <= 0.5
%          power1 = 1000;
%          power2 = 1000;
%          power3 = 0;
%          v1 = 2;
%          v2 = 1; 
%         else
%             if deltaT <= 1
%                 power1 = 1000;
%                 power2 = 0;
%                 power3 = 0;
%                 v1 = 2;
%                 v2 = 1;
%             else
%                 power1 = 0;
%                 power2 = 0;
%                 power3 = 0;
%                 v1 = 0;
%                 v2 = 0;
%             end
%         end

%       if power == 0
%           v1 = 0;
%           v2 = 0;
%       else
%           v1 = 2;
%           v2 = 1;
%       end
% 
%     end
% 
% end

== matlab function NewKitchen_demo/Motion detection3/MATLAB Function ==
  data: num input; signal output
function signal = motion(num)
    
    N = ceil(num/30); 
    
    if N == 1
        signal = 1; % 5 + 3
    elseif N == 2
        signal = 1; % 3 + 3
    elseif N == 3
        signal = 1; % 2 + 3
    elseif N == 4
        signal = 1; % 7 + 3
    elseif N == 5
        signal = 1; % 6 + 3
    elseif N == 6
        signal = 1; % 4 + 3
    else
        signal = 1;
    end
    
end

== stateflow chart NewKitchen_demo/EMS2 ==
  state OFF_Mode
    during:
    power = 0;
  state ON_Mode
    state Mode3
      during:
      power = 3300;
    (default) -> Mode3
  (default) -> (junction 1)
  (junction 1) -> OFF_Mode [order 1] : [T>=24]
  (junction 1) -> ON_Mode [order 2]
  OFF_Mode -> ON_Mode : [T<22]
  ON_Mode -> OFF_Mode : [T>=23]
  data: T input; power output

== stateflow chart NewKitchen_demo/EMS3 ==
  state OFF_Mode
    during:
    power = 0;
  state ON_Mode
    state Mode1
      during:
      power = 1100;
    state Mode2
      during:
      power = 2200;
    state Mode3
      during:
      power = 3300;
    (default) -> Mode3
    Mode3 -> Mode2 : [T>23]
    Mode2 -> Mode1 : [T>23.7]
  (default) -> (junction 1)
  (junction 1) -> OFF_Mode [order 1] : [T>=24]
  (junction 1) -> ON_Mode [order 2]
  OFF_Mode -> ON_Mode : [T<22]
  ON_Mode -> OFF_Mode : [T>=24]
  data: T input; power output

== matlab function NewKitchen_demo/MATLAB Function1 ==
  data: power1 output; power2 output; power3 output; num input; v1 output; v2 output
function [power1,power2,power3,v1,v2] = motion(num)
    
    N = ceil(num/10); 

    if N <= 1
        power1 = 1000;
        power2 = 1000;
        power3 = 1000;
        v1 = 0;
        v2 = 0;
    else

        if N <= 2
         power1 = 0;
         power2 = 0;
         power3 = 0;
         v1 = 3;
         v2 = 1; 
        else
         power1 = 0;
         power2 = 0;
         power3 = 0;
         v1 = 0;
         v2 = 0; 
        end

%       if power == 0
%           v1 = 0;
%           v2 = 0;
%       else
%           v1 = 2;
%           v2 = 1;
%       end

    end

end

== stateflow chart NewKitchen_demo/EMS4 ==
  state OFF_Mode
    power1 = 0;
    power2 = 0;
    power3 = 0;
    v1 = 0;
    v2 = 0;
  state ON_Mode
    state Mode1
      state Mode1off
        power1 = 0;
        power2 = 0;
        power3 = 0;
        v1 = 2;
        v2 = 1;
      state Mode1on
        power1 = 1000;
        power2 = 0;
        power3 = 0;
        v1 = 2;
        v2 = 1;
      (default) -> Mode1on
      Mode1on -> Mode1off : [deltaT>=0.03]
      Mode1off -> Mode1on : [deltaT<0.03]
    state Mode3
      state Mode3off
        power1 = 0;
        power2 = 0;
        power3 = 0;
        v1 = 2;
        v2 = 1;
      state Mode3on
        power1 = 1000;
        power2 = 1000;
        power3 = 1000;
        v1 = 2;
        v2 = 1;
      (default) -> Mode3on
      Mode3on -> Mode3off : [deltaT>=0.12]
      Mode3off -> Mode3on : [deltaT<0.12]
    state Mode2
      state Mode2off
        power1 = 0;
        power2 = 0;
        power3 = 0;
        v1 = 2;
        v2 = 1;
      state Mode2on
        power1 = 1000;
        power2 = 1000;
        power3 = 0;
        v1 = 2;
        v2 = 1;
      (default) -> Mode2on
      Mode2on -> Mode2off : [deltaT>=0.06]
      Mode2off -> Mode2on : [deltaT<0.06]
    (junction 6) -> Mode2 [order 2]
    (default) -> (junction 6)
    (junction 6) -> Mode3 [order 1] : [T<=21.5]
    Mode1 -> Mode3 [order 2] : [deltaT<0]
    Mode2 -> Mode3 [order 2] : [deltaT<=0.02]
    Mode3 -> Mode1 : [T>22.5&deltaT>0.03]
    Mode2 -> Mode1 [order 1] : [T>22.5&deltaT>0.03]
    Mode1 -> Mode2 [order 1] : [deltaT<=0.015&deltaT>=0]
  (default) -> (junction 1)
  (junction 1) -> OFF_Mode [order 1] : [T>=23]
  (junction 1) -> ON_Mode [order 2]
  OFF_Mode -> ON_Mode : [T<22]
  ON_Mode -> OFF_Mode : [T>=23]
  data: T input; power1 output; deltaT input; power2 output; power3 output; v1 output; v2 output

== matlab function NewKitchen_demo/Subsystem5/MATLAB Function ==
  data: num input; signal output
function signal = motion(num)
    
    N = ceil(num/30); 
    
    if N == 1
        signal = 1; % 6 + 3
    else
        signal = 2;
    end
    
end

== matlab function NewKitchen_demo/Motion detection1/MATLAB Function ==
  data: num input; signal output
function signal = motion(num)
    
    N = ceil(num/30); 
    
    if N == 1
        signal = 6 + 3;
    elseif N == 2
        signal = 3 + 3;
    elseif N == 3
        signal = 7 + 3;
    elseif N == 4
        signal = 12;
    elseif N == 5
        signal = 8 + 3;
    elseif N == 6
        signal = 5 + 3;
    elseif N == 7
        signal = 12;
    elseif N == 8
        signal = 12;
    elseif N == 9
        signal = 2 + 3;
    elseif N == 10
        signal = 4 + 3;
    else
        signal = 0;
    end
    
end

== stateflow chart NewKitchen_demo/EMS1 ==
  state OFF_Mode
    during:
    power = 0;
  state ON_Mode
    state Mode1
      during:
      power = 1100;
    state Mode2
      during:
      power = 2200;
    state Mode3
      during:
      power = 3300;
    (default) -> (junction 6)
    (junction 6) -> Mode3 [order 2]
    (junction 6) -> Mode2 [order 1] : [T>=22]
    Mode2 -> Mode1 : [T>23.5]
    Mode3 -> Mode1 : [T>23.5]
  (default) -> (junction 1)
  (junction 1) -> OFF_Mode [order 1] : [T>=24]
  (junction 1) -> ON_Mode [order 2]
  OFF_Mode -> ON_Mode : [T<22]
  ON_Mode -> OFF_Mode : [T>=24]
  data: T input; power output
